simulink model "ME425QuadcoptorMotionControlV4"  (R2024b)
settings: Solver=VariableStepAuto  StartTime=0.0  StopTime=simTime  FixedStep=1e-9  RelTol=1e-2
values from neighbouring files (symbols this model uses):
  D_phi = 0.95    [ME425HW3QuadcoptorMotionControl.m]
  D_psi = 0.95    [ME425HW3QuadcoptorMotionControl.m]
  D_theta = 0.95    [ME425HW3QuadcoptorMotionControl.m]
  D_z = 2    [ME425HW3QuadcoptorMotionControl.m]
  g = 9.81    [ME425HW3QuadcoptorMotionControl.m]
  I_phi = 0.1    [ME425HW3QuadcoptorMotionControl.m]
  I_psi = 0.05    [ME425HW3QuadcoptorMotionControl.m]
  I_theta = 0.1    [ME425HW3QuadcoptorMotionControl.m]
  I_z = 0.1    [ME425HW3QuadcoptorMotionControl.m]
  initialAngles = [0 0 0]    [ME425HW3QuadcoptorMotionControl.m]
  Ix = 0.02    [ME425HW3QuadcoptorMotionControl.m]
  Iy = 0.02    [ME425HW3QuadcoptorMotionControl.m]
  Iz = 0.04    [ME425HW3QuadcoptorMotionControl.m]
  m = 1    [ME425HW3QuadcoptorMotionControl.m]
  P_phi = 0.5    [ME425HW3QuadcoptorMotionControl.m]
  P_psi = 0.5    [ME425HW3QuadcoptorMotionControl.m]
  P_theta = 0.5    [ME425HW3QuadcoptorMotionControl.m]
  P_z = 0.75    [ME425HW3QuadcoptorMotionControl.m]
  zDesired = 2    [ME425HW3QuadcoptorMotionControl.m]
libraries: slpidlib x4
settings Model: Creator=Arda Gencer  LastModifiedBy=Arda Gencer

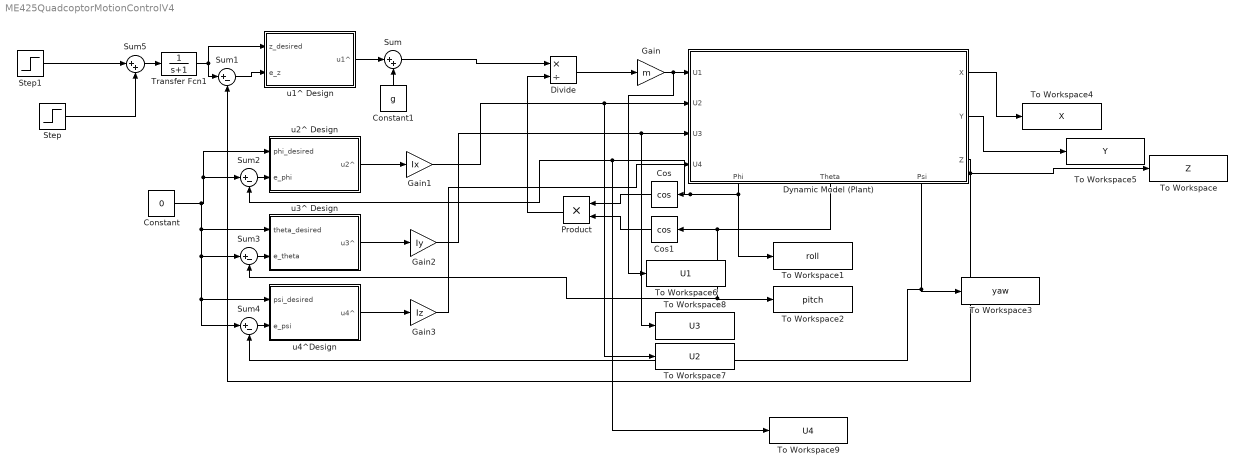
== system ME425QuadcoptorMotionControlV4 ==
  Constant : Constant  Value=0
  Constant1 : Constant  Value=g
  Cos : Trigonometry  Operator=cos
  Cos1 : Trigonometry  Operator=cos
  Divide : Product  Inputs=*/
  Dynamic Model (Plant) : Subsystem
      settings: PortSchema="{\"entries\":[{\"content\":{\"sides\":[{\"content\":{\"connectorIds\":[\"In1\",\"In2\",\"In3\",\"In4\"]},\"type\":\"ConnectorPlacement.EquallySpacedRectSide\",\"uuid\":\"08b1677c-733e-4bff-a275-c4be774b24b5\"},{\"content\":{\"connectorIds\":[\"Out1\",\"Out2\",\"Out3\"],\"side\":\"RIGHT\"},\"type\":\"ConnectorPlacement.EquallySpacedRectSide\",\"uuid\":\"655169e1-9348-4dc0-9050-0d096e576661\"},{\"content\":{\"side\":\"TOP\"},\"type\":\"ConnectorPlacement.EquallySpacedRectSide\",\"uuid\":\"6c01dbd3-88d9-43d1-9966-b2f3dc36f972\"},{\"content\":{\"connectorIds\":[\"Out4\",\"Out5\",\"Out6\"],\"side\":\"BOTTOM\"},\"type\":\"ConnectorPlacement.EquallySpacedRectSide\",\"uuid\":\"d00d5ad9-d72f-434d-885b-77b5f35ca427\"}]},\"type\":\"ConnectorPlacement.EquallySpacedConnector\",\"uuid\":\"87e83324-135b-4426-b2c1-a0cfdb552e41\"}],\"packageUris\":[\"http://schema.mathworks.com/mf0/Connector/R2020b\"],\"version\":\"1.0\"}"
  Gain : Gain  Gain=m
  Gain1 : Gain  Gain=Ix
  Gain2 : Gain  Gain=Iy
  Gain3 : Gain  Gain=Iz
  Product : Product
  Step : Step  Time=0  After=zDesired  SampleTime=0
  Step1 : Step  Time=30  After=-zDesired  SampleTime=0
  Sum : Sum  Inputs=|++
  Sum{1..4} (4 alike) : Sum  Inputs=|+-
  Sum5 : Sum  Inputs=|++
  To Workspace : ToWorkspace  VariableName=Z  SampleTime=-1
  To Workspace1 : ToWorkspace  VariableName=roll  SampleTime=-1
  To Workspace2 : ToWorkspace  VariableName=pitch  SampleTime=-1
  To Workspace3 : ToWorkspace  VariableName=yaw  SampleTime=-1
  To Workspace4 : ToWorkspace  VariableName=X  SampleTime=-1
  To Workspace5 : ToWorkspace  VariableName=Y  SampleTime=-1
  To Workspace6 : ToWorkspace  VariableName=U1  SampleTime=-1
  To Workspace7 : ToWorkspace  VariableName=U2  SampleTime=-1
  To Workspace8 : ToWorkspace  VariableName=U3  SampleTime=-1
  To Workspace9 : ToWorkspace  VariableName=U4  SampleTime=-1
  Transfer Fcn1 : TransferFcn  Denominator=[1 1]
  u1^ Design : Subsystem
  u2^ Design : Subsystem
  u3^ Design : Subsystem
  u4^Design : Subsystem
  wires:
  Dynamic Model (Plant)/3(Z) -> Sum1/2, To Workspace/1
  Dynamic Model (Plant)/4(Phi) -> To Workspace1/1, To Workspace9/1, Sum2/2, Cos/1
  Dynamic Model (Plant)/5(Theta) -> Sum3/2, To Workspace2/1, Cos1/1
  Dynamic Model (Plant)/6(Psi) -> Sum4/2, To Workspace3/1
  Transfer Fcn1/1 -> u1^ Design/1(z_desired), Sum1/1
  Constant1/1 -> Sum/2
  Gain/1 -> To Workspace6/1, Dynamic Model (Plant)/1(U1)
  Divide/1 -> Gain/1
  Product/1 -> Divide/2
  Sum/1 -> Divide/1
  Cos/1 -> Product/1
  Cos1/1 -> Product/2
  u1^ Design/1(u1^) -> Sum/1
  Sum1/1 -> u1^ Design/2(e_z)
  Constant/1 -> Sum4/1, u4^Design/1(psi_desired), Sum3/1, u3^ Design/1(theta_desired), Sum2/1, u2^ Design/1(phi_desired)
  Sum4/1 -> u4^Design/2(e_psi)
  Sum3/1 -> u3^ Design/2(e_theta)
  Sum2/1 -> u2^ Design/2(e_phi)
  u2^ Design/1(u2^) -> Gain1/1
  u4^Design/1(u4^) -> Gain3/1
  u3^ Design/1(u3^) -> Gain2/1
  Gain1/1 -> To Workspace7/1, Dynamic Model (Plant)/2(U2)
  Gain2/1 -> Dynamic Model (Plant)/3(U3), To Workspace8/1
  Gain3/1 -> Dynamic Model (Plant)/4(U4)
  Step1/1 -> Sum5/1
  Step/1 -> Sum5/2
  Dynamic Model (Plant)/1(X) -> To Workspace4/1
  Dynamic Model (Plant)/2(Y) -> To Workspace5/1
  Sum5/1 -> Transfer Fcn1/1

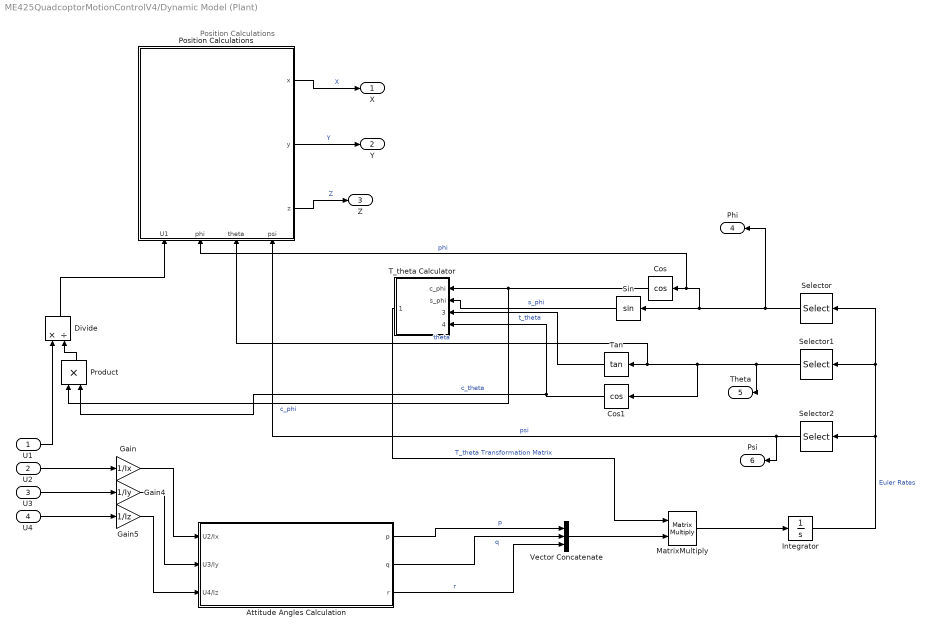
== system ME425QuadcoptorMotionControlV4/Dynamic Model (Plant) ==
  note: Position Calculations
  U1 : Inport
  U2 : Inport  Port=2
  U3 : Inport  Port=3
  U4 : Inport  Port=4
  Attitude Angles Calculation : Subsystem
  Cos : Trigonometry  Operator=cos
  Cos1 : Trigonometry  Operator=cos
  Divide : Product  Inputs=*/
  Gain : Gain  Gain=1/Ix
  Gain4 : Gain  Gain=1/Iy
  Gain5 : Gain  Gain=1/Iz
  Integrator : Integrator  InitialCondition=initialAngles
  MatrixMultiply : Product  Multiplication=Matrix(*)
  Position Calculations : Subsystem
      settings: PortSchema="{\"entries\":[{\"content\":{\"sides\":[{\"content\":{\"connectorIds\":[\"In1\",\"In2\",\"In3\",\"In4\"]},\"type\":\"ConnectorPlacement.EquallySpacedRectSide\",\"uuid\":\"bd898587-7085-4c8a-abc4-67bd8d59ea08\"},{\"content\":{\"side\":\"RIGHT\"},\"type\":\"ConnectorPlacement.EquallySpacedRectSide\",\"uuid\":\"f25e6be6-ac4f-428e-a4d0-66b7114170c6\"},{\"content\":{\"side\":\"TOP\"},\"type\":\"ConnectorPlacement.EquallySpacedRectSide\",\"uuid\":\"1b5079d3-453d-4b69-91fa-2e9092c60c78\"},{\"content\":{\"connectorIds\":[\"Out1\",\"Out2\",\"Out3\"],\"side\":\"BOTTOM\"},\"type\":\"ConnectorPlacement.EquallySpacedRectSide\",\"uuid\":\"956a8f80-6aeb-4d85-a1cd-c5deb734e20d\"}]},\"type\":\"ConnectorPlacement.EquallySpacedConnector\",\"uuid\":\"f46b91c2-157f-4b6c-9de1-eab5cbe73704\"}],\"packageUris\":[\"http://schema.mathworks.com/mf0/Connector/R2020b\"],\"version\":\"1.0\"}"
  Product : Product
  Selector : Selector  InputPortWidth=3  IndexOptions=Index vector (dialog)  Indices=[1]  OutputSizes=1
  Selector1 : Selector  InputPortWidth=3  IndexOptions=Index vector (dialog)  Indices=2  OutputSizes=1
  Selector2 : Selector  InputPortWidth=3  IndexOptions=Index vector (dialog)  Indices=3  OutputSizes=1
  Sin : Trigonometry
  T_theta Calculator : Subsystem
  Tan : Trigonometry  Operator=tan
  Vector Concatenate : Concatenate  NumInputs=3
  X : Outport
  Y : Outport  Port=2
  Z : Outport  Port=3
  Phi : Outport  Port=4
  Theta : Outport  Port=5
  Psi : Outport  Port=6
  wires:
  Vector Concatenate/1 -> MatrixMultiply/2
  Selector1/1 -> Theta/1, Position Calculations/3(theta), Tan/1, Cos1/1  "theta"
  Attitude Angles Calculation/2(q) -> Vector Concatenate/2  "q"
  U4/1 -> Gain5/1
  Cos/1 -> Product/1, T_theta Calculator/1(c_phi)  "c_phi"
  Selector/1 -> Phi/1, Position Calculations/2(phi), Cos/1, Sin/1  "phi"
  Gain/1 -> Attitude Angles Calculation/1(U2/Ix)
  Gain5/1 -> Attitude Angles Calculation/3(U4/Iz)
  Attitude Angles Calculation/3(r) -> Vector Concatenate/3  "r"
  Tan/1 -> T_theta Calculator/3(t_theta)  "t_theta"
  Sin/1 -> T_theta Calculator/2(s_phi)  "s_phi"
  Cos1/1 -> Product/2, T_theta Calculator/4(c_theta)  "c_theta"
  MatrixMultiply/1 -> Integrator/1
  T_theta Calculator/1(T_theta) -> MatrixMultiply/1  "T_theta Transformation Matrix"
  U2/1 -> Gain/1
  U3/1 -> Gain4/1
  Selector2/1 -> Psi/1, Position Calculations/4(psi)  "psi"
  Attitude Angles Calculation/1(p) -> Vector Concatenate/1  "p"
  Position Calculations/1(z) -> Z/1  "Z"
  Gain4/1 -> Attitude Angles Calculation/2(U3/Iy)
  Position Calculations/3(x) -> X/1  "X"
  Position Calculations/2(y) -> Y/1  "Y"
  U1/1 -> Divide/1
  Divide/1 -> Position Calculations/1(U1)
  Product/1 -> Divide/2
  Integrator/1 -> Selector/1, Selector1/1, Selector2/1  "Euler Rates"

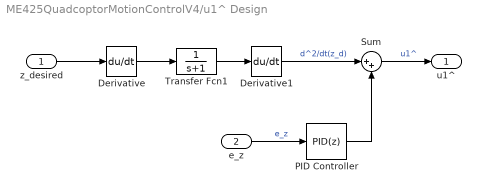
== system ME425QuadcoptorMotionControlV4/u1^ Design ==
  z_desired : Inport
  e_z : Inport  Port=2
  Derivative : Derivative
  Derivative1 : Derivative
  PID Controller : slpidlib/PID Controller  Controller=PID  Form=Parallel  TimeDomain=Discrete-time  UseExternalTs=off  SampleTime=0.001  IntegratorMethod=Forward Euler  FilterMethod=Forward Euler  ControllerParametersSource=internal  P=P_z  I=I_z  UseKiTs=off  D=D_z  UseExternalDerivativeSource=off  N=100  UseFilter=on  TunerSelectOption=Transfer Function Based (PID Tuner App)  InitialConditionSource=internal  InitialConditionForIntegrator=0  InitialConditionForFilter=0  DifferentiatorICPrevScaledInput=0  ExternalReset=none  TrackingMode=off  Kt=1  LimitOutput=off  SatLimitsSource=internal  UpperSaturationLimit=inf  LowerSaturationLimit=-inf  LinearizeAsGain=on  AntiWindupMode=none  Kb=1  LimitIntegrator=off  UpperIntegratorSaturationLimit=inf  LowerIntegratorSaturationLimit=-inf  POutMin=[]  POutMax=[]  IOutMin=[]  IOutMax=[]  DOutMin=[]  DOutMax=[]  NOutMin=[]  NOutMax=[]  SumOutMin=[]  SumOutMax=[]  SaturationOutMin=[]  SaturationOutMax=[]  PParamMin=[]  PParamMax=[]  IParamMin=[]  IParamMax=[]  DParamMin=[]  DParamMax=[]  NParamMin=[]  NParamMax=[]  KbParamMin=[]  KbParamMax=[]  KtParamMin=[]  KtParamMax=[]  KbOutMin=[]  KbOutMax=[]  KtOutMin=[]  KtOutMax=[]  IntegratorOutMin=[]  IntegratorOutMax=[]  FilterOutMin=[]  FilterOutMax=[]  SumI1OutMin=[]  SumI1OutMax=[]  SumI2OutMin=[]  SumI2OutMax=[]  SumI3OutMin=[]  SumI3OutMax=[]  SumI4OutMin=[]  SumI4OutMax=[]  SumDOutMin=[]  SumDOutMax=[]  DifferentiatorOutMin=[]  DifferentiatorOutMax=[]  FilterDiffOutCoefMin=[]  FilterDiffOutCoefMax=[]  ReciprocalOutMin=[]  ReciprocalOutMax=[]  SumDenOutMin=[]  SumDenOutMax=[]  SumNumOutMin=[]  SumNumOutMax=[]  DivideOutMin=[]  DivideOutMax=[]  UdiffTsProdOutMin=[]  UdiffTsProdOutMax=[]  NTsProdOutMin=[]  NTsProdOutMax=[]  UintegralTsProdOutMin=[]  UintegralTsProdOutMax=[]  UngainTsProdOutMin=[]  UngainTsProdOutMax=[]  ClampingZeroOutDataTypeStr=Inherit: Inherit via back propagation  ClampingZeroOutMin=[]  ClampingZeroOutMax=[]  FilterDenConstantOutDataTypeStr=Inherit: Inherit via back propagation  FilterDenConstantOutMin=[]  FilterDenConstantOutMax=[]  PCopyOutDataTypeStr=Inherit: Inherit via back propagation  PCopyOutMin=[]  PCopyOutMax=[]  NCopyOutDataTypeStr=Inherit: Inherit via back propagation  NCopyOutMin=[]  NCopyOutMax=[]  IntegratorContinuousStateAttributes=''  IntegratorStateMustResolveToSignalObject=off  IntegratorRTWStateStorageClass=Auto  FilterContinuousStateAttributes=''  FilterStateMustResolveToSignalObject=off  FilterRTWStateStorageClass=Auto  ParallelPVariant=InternalParameters  IdealPVariant=Disabled  IVariant=InternalParameters  DVariant=InternalParameters  IntegratorVariant=Discrete  SatVariant=Disabled  AWVariant=Passthrough  PCopyVariant=Disabled  TRVariant=Disabled  FdbkBlocksVariant=Forward  IdealPFdbkVariant=Disabled  SatFdbkVariant=Disabled  DerivativeFilterVariant=ForwardEulerFilter  NVariant=InternalParameters  NCopyVariant=Disabled  FilterICVariant=InternalICsFilter  IntegratorICVariant=InternalICs  ExternalResetVariant=Disabled  TRSumVariant=Passthrough  SumFdbkVariant=Disabled  SumVariant=Sum_PID  TsampFilterVariant=InternalTs  TsampNgainVariant=Passthrough  TsampIntegralVariant=Disabled_SignalSpec  ExternalSaturationOutDataTypeStr=Inherit: Same as second input  DerivativeSourceVariant=ErrorSignal  PreIntVariant=InternalPreInt
  Sum : Sum  Inputs=|++
  Transfer Fcn1 : TransferFcn  Denominator=[1 1]
  u1^ : Outport
  wires:
  z_desired/1 -> Derivative/1
  Derivative1/1 -> Sum/1  "d^2/dt(z_d)"
  Derivative/1 -> Transfer Fcn1/1
  PID Controller/1 -> Sum/2
  e_z/1 -> PID Controller/1  "e_z"
  Sum/1 -> u1^/1  "u1^"
  Transfer Fcn1/1 -> Derivative1/1

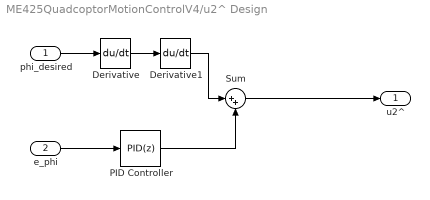
== system ME425QuadcoptorMotionControlV4/u2^ Design ==
  phi_desired : Inport
  e_phi : Inport  Port=2
  Derivative : Derivative
  Derivative1 : Derivative
  PID Controller : slpidlib/PID Controller  Controller=PID  Form=Parallel  TimeDomain=Discrete-time  UseExternalTs=off  SampleTime=0.001  IntegratorMethod=Forward Euler  FilterMethod=Forward Euler  ControllerParametersSource=internal  P=P_phi  I=I_phi  UseKiTs=off  D=D_phi  UseExternalDerivativeSource=off  N=100  UseFilter=on  TunerSelectOption=Transfer Function Based (PID Tuner App)  InitialConditionSource=internal  InitialConditionForIntegrator=0  InitialConditionForFilter=0  DifferentiatorICPrevScaledInput=0  ExternalReset=none  TrackingMode=off  Kt=1  LimitOutput=off  SatLimitsSource=internal  UpperSaturationLimit=inf  LowerSaturationLimit=-inf  LinearizeAsGain=on  AntiWindupMode=none  Kb=1  LimitIntegrator=off  UpperIntegratorSaturationLimit=inf  LowerIntegratorSaturationLimit=-inf  POutMin=[]  POutMax=[]  IOutMin=[]  IOutMax=[]  DOutMin=[]  DOutMax=[]  NOutMin=[]  NOutMax=[]  SumOutMin=[]  SumOutMax=[]  SaturationOutMin=[]  SaturationOutMax=[]  PParamMin=[]  PParamMax=[]  IParamMin=[]  IParamMax=[]  DParamMin=[]  DParamMax=[]  NParamMin=[]  NParamMax=[]  KbParamMin=[]  KbParamMax=[]  KtParamMin=[]  KtParamMax=[]  KbOutMin=[]  KbOutMax=[]  KtOutMin=[]  KtOutMax=[]  IntegratorOutMin=[]  IntegratorOutMax=[]  FilterOutMin=[]  FilterOutMax=[]  SumI1OutMin=[]  SumI1OutMax=[]  SumI2OutMin=[]  SumI2OutMax=[]  SumI3OutMin=[]  SumI3OutMax=[]  SumI4OutMin=[]  SumI4OutMax=[]  SumDOutMin=[]  SumDOutMax=[]  DifferentiatorOutMin=[]  DifferentiatorOutMax=[]  FilterDiffOutCoefMin=[]  FilterDiffOutCoefMax=[]  ReciprocalOutMin=[]  ReciprocalOutMax=[]  SumDenOutMin=[]  SumDenOutMax=[]  SumNumOutMin=[]  SumNumOutMax=[]  DivideOutMin=[]  DivideOutMax=[]  UdiffTsProdOutMin=[]  UdiffTsProdOutMax=[]  NTsProdOutMin=[]  NTsProdOutMax=[]  UintegralTsProdOutMin=[]  UintegralTsProdOutMax=[]  UngainTsProdOutMin=[]  UngainTsProdOutMax=[]  ClampingZeroOutDataTypeStr=Inherit: Inherit via back propagation  ClampingZeroOutMin=[]  ClampingZeroOutMax=[]  FilterDenConstantOutDataTypeStr=Inherit: Inherit via back propagation  FilterDenConstantOutMin=[]  FilterDenConstantOutMax=[]  PCopyOutDataTypeStr=Inherit: Inherit via back propagation  PCopyOutMin=[]  PCopyOutMax=[]  NCopyOutDataTypeStr=Inherit: Inherit via back propagation  NCopyOutMin=[]  NCopyOutMax=[]  IntegratorContinuousStateAttributes=''  IntegratorStateMustResolveToSignalObject=off  IntegratorRTWStateStorageClass=Auto  FilterContinuousStateAttributes=''  FilterStateMustResolveToSignalObject=off  FilterRTWStateStorageClass=Auto  ParallelPVariant=InternalParameters  IdealPVariant=Disabled  IVariant=InternalParameters  DVariant=InternalParameters  IntegratorVariant=Discrete  SatVariant=Disabled  AWVariant=Passthrough  PCopyVariant=Disabled  TRVariant=Disabled  FdbkBlocksVariant=Forward  IdealPFdbkVariant=Disabled  SatFdbkVariant=Disabled  DerivativeFilterVariant=ForwardEulerFilter  NVariant=InternalParameters  NCopyVariant=Disabled  FilterICVariant=InternalICsFilter  IntegratorICVariant=InternalICs  ExternalResetVariant=Disabled  TRSumVariant=Passthrough  SumFdbkVariant=Disabled  SumVariant=Sum_PID  TsampFilterVariant=InternalTs  TsampNgainVariant=Passthrough  TsampIntegralVariant=Disabled_SignalSpec  ExternalSaturationOutDataTypeStr=Inherit: Same as second input  DerivativeSourceVariant=ErrorSignal  PreIntVariant=InternalPreInt
  Sum : Sum  Inputs=|++
  u2^ : Outport
  wires:
  phi_desired/1 -> Derivative/1
  Derivative/1 -> Derivative1/1
  e_phi/1 -> PID Controller/1
  Derivative1/1 -> Sum/1
  PID Controller/1 -> Sum/2
  Sum/1 -> u2^/1

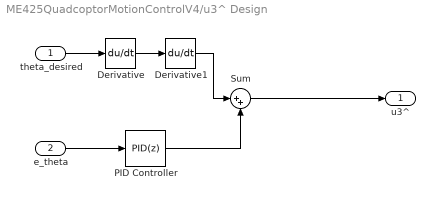
== system ME425QuadcoptorMotionControlV4/u3^ Design ==
  theta_desired : Inport
  e_theta : Inport  Port=2
  Derivative : Derivative
  Derivative1 : Derivative
  PID Controller : slpidlib/PID Controller  Controller=PID  Form=Parallel  TimeDomain=Discrete-time  UseExternalTs=off  SampleTime=0.001  IntegratorMethod=Forward Euler  FilterMethod=Forward Euler  ControllerParametersSource=internal  P=P_theta  I=I_theta  UseKiTs=off  D=D_theta  UseExternalDerivativeSource=off  N=100  UseFilter=on  TunerSelectOption=Transfer Function Based (PID Tuner App)  InitialConditionSource=internal  InitialConditionForIntegrator=0  InitialConditionForFilter=0  DifferentiatorICPrevScaledInput=0  ExternalReset=none  TrackingMode=off  Kt=1  LimitOutput=off  SatLimitsSource=internal  UpperSaturationLimit=inf  LowerSaturationLimit=-inf  LinearizeAsGain=on  AntiWindupMode=none  Kb=1  LimitIntegrator=off  UpperIntegratorSaturationLimit=inf  LowerIntegratorSaturationLimit=-inf  POutMin=[]  POutMax=[]  IOutMin=[]  IOutMax=[]  DOutMin=[]  DOutMax=[]  NOutMin=[]  NOutMax=[]  SumOutMin=[]  SumOutMax=[]  SaturationOutMin=[]  SaturationOutMax=[]  PParamMin=[]  PParamMax=[]  IParamMin=[]  IParamMax=[]  DParamMin=[]  DParamMax=[]  NParamMin=[]  NParamMax=[]  KbParamMin=[]  KbParamMax=[]  KtParamMin=[]  KtParamMax=[]  KbOutMin=[]  KbOutMax=[]  KtOutMin=[]  KtOutMax=[]  IntegratorOutMin=[]  IntegratorOutMax=[]  FilterOutMin=[]  FilterOutMax=[]  SumI1OutMin=[]  SumI1OutMax=[]  SumI2OutMin=[]  SumI2OutMax=[]  SumI3OutMin=[]  SumI3OutMax=[]  SumI4OutMin=[]  SumI4OutMax=[]  SumDOutMin=[]  SumDOutMax=[]  DifferentiatorOutMin=[]  DifferentiatorOutMax=[]  FilterDiffOutCoefMin=[]  FilterDiffOutCoefMax=[]  ReciprocalOutMin=[]  ReciprocalOutMax=[]  SumDenOutMin=[]  SumDenOutMax=[]  SumNumOutMin=[]  SumNumOutMax=[]  DivideOutMin=[]  DivideOutMax=[]  UdiffTsProdOutMin=[]  UdiffTsProdOutMax=[]  NTsProdOutMin=[]  NTsProdOutMax=[]  UintegralTsProdOutMin=[]  UintegralTsProdOutMax=[]  UngainTsProdOutMin=[]  UngainTsProdOutMax=[]  ClampingZeroOutDataTypeStr=Inherit: Inherit via back propagation  ClampingZeroOutMin=[]  ClampingZeroOutMax=[]  FilterDenConstantOutDataTypeStr=Inherit: Inherit via back propagation  FilterDenConstantOutMin=[]  FilterDenConstantOutMax=[]  PCopyOutDataTypeStr=Inherit: Inherit via back propagation  PCopyOutMin=[]  PCopyOutMax=[]  NCopyOutDataTypeStr=Inherit: Inherit via back propagation  NCopyOutMin=[]  NCopyOutMax=[]  IntegratorContinuousStateAttributes=''  IntegratorStateMustResolveToSignalObject=off  IntegratorRTWStateStorageClass=Auto  FilterContinuousStateAttributes=''  FilterStateMustResolveToSignalObject=off  FilterRTWStateStorageClass=Auto  ParallelPVariant=InternalParameters  IdealPVariant=Disabled  IVariant=InternalParameters  DVariant=InternalParameters  IntegratorVariant=Discrete  SatVariant=Disabled  AWVariant=Passthrough  PCopyVariant=Disabled  TRVariant=Disabled  FdbkBlocksVariant=Forward  IdealPFdbkVariant=Disabled  SatFdbkVariant=Disabled  DerivativeFilterVariant=ForwardEulerFilter  NVariant=InternalParameters  NCopyVariant=Disabled  FilterICVariant=InternalICsFilter  IntegratorICVariant=InternalICs  ExternalResetVariant=Disabled  TRSumVariant=Passthrough  SumFdbkVariant=Disabled  SumVariant=Sum_PID  TsampFilterVariant=InternalTs  TsampNgainVariant=Passthrough  TsampIntegralVariant=Disabled_SignalSpec  ExternalSaturationOutDataTypeStr=Inherit: Same as second input  DerivativeSourceVariant=ErrorSignal  PreIntVariant=InternalPreInt
  Sum : Sum  Inputs=|++
  u3^ : Outport
  wires:
  theta_desired/1 -> Derivative/1
  Derivative/1 -> Derivative1/1
  e_theta/1 -> PID Controller/1
  Derivative1/1 -> Sum/1
  PID Controller/1 -> Sum/2
  Sum/1 -> u3^/1

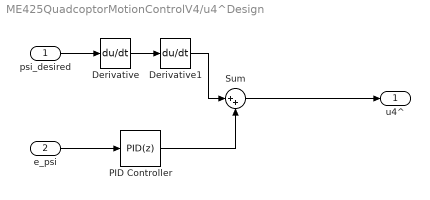
== system ME425QuadcoptorMotionControlV4/u4^Design ==
  psi_desired : Inport
  e_psi : Inport  Port=2
  Derivative : Derivative
  Derivative1 : Derivative
  PID Controller : slpidlib/PID Controller  Controller=PID  Form=Parallel  TimeDomain=Discrete-time  UseExternalTs=off  SampleTime=0.001  IntegratorMethod=Forward Euler  FilterMethod=Forward Euler  ControllerParametersSource=internal  P=P_psi  I=I_psi  UseKiTs=off  D=D_psi  UseExternalDerivativeSource=off  N=100  UseFilter=on  TunerSelectOption=Transfer Function Based (PID Tuner App)  InitialConditionSource=internal  InitialConditionForIntegrator=0  InitialConditionForFilter=0  DifferentiatorICPrevScaledInput=0  ExternalReset=none  TrackingMode=off  Kt=1  LimitOutput=off  SatLimitsSource=internal  UpperSaturationLimit=inf  LowerSaturationLimit=-inf  LinearizeAsGain=on  AntiWindupMode=none  Kb=1  LimitIntegrator=off  UpperIntegratorSaturationLimit=inf  LowerIntegratorSaturationLimit=-inf  POutMin=[]  POutMax=[]  IOutMin=[]  IOutMax=[]  DOutMin=[]  DOutMax=[]  NOutMin=[]  NOutMax=[]  SumOutMin=[]  SumOutMax=[]  SaturationOutMin=[]  SaturationOutMax=[]  PParamMin=[]  PParamMax=[]  IParamMin=[]  IParamMax=[]  DParamMin=[]  DParamMax=[]  NParamMin=[]  NParamMax=[]  KbParamMin=[]  KbParamMax=[]  KtParamMin=[]  KtParamMax=[]  KbOutMin=[]  KbOutMax=[]  KtOutMin=[]  KtOutMax=[]  IntegratorOutMin=[]  IntegratorOutMax=[]  FilterOutMin=[]  FilterOutMax=[]  SumI1OutMin=[]  SumI1OutMax=[]  SumI2OutMin=[]  SumI2OutMax=[]  SumI3OutMin=[]  SumI3OutMax=[]  SumI4OutMin=[]  SumI4OutMax=[]  SumDOutMin=[]  SumDOutMax=[]  DifferentiatorOutMin=[]  DifferentiatorOutMax=[]  FilterDiffOutCoefMin=[]  FilterDiffOutCoefMax=[]  ReciprocalOutMin=[]  ReciprocalOutMax=[]  SumDenOutMin=[]  SumDenOutMax=[]  SumNumOutMin=[]  SumNumOutMax=[]  DivideOutMin=[]  DivideOutMax=[]  UdiffTsProdOutMin=[]  UdiffTsProdOutMax=[]  NTsProdOutMin=[]  NTsProdOutMax=[]  UintegralTsProdOutMin=[]  UintegralTsProdOutMax=[]  UngainTsProdOutMin=[]  UngainTsProdOutMax=[]  ClampingZeroOutDataTypeStr=Inherit: Inherit via back propagation  ClampingZeroOutMin=[]  ClampingZeroOutMax=[]  FilterDenConstantOutDataTypeStr=Inherit: Inherit via back propagation  FilterDenConstantOutMin=[]  FilterDenConstantOutMax=[]  PCopyOutDataTypeStr=Inherit: Inherit via back propagation  PCopyOutMin=[]  PCopyOutMax=[]  NCopyOutDataTypeStr=Inherit: Inherit via back propagation  NCopyOutMin=[]  NCopyOutMax=[]  IntegratorContinuousStateAttributes=''  IntegratorStateMustResolveToSignalObject=off  IntegratorRTWStateStorageClass=Auto  FilterContinuousStateAttributes=''  FilterStateMustResolveToSignalObject=off  FilterRTWStateStorageClass=Auto  ParallelPVariant=InternalParameters  IdealPVariant=Disabled  IVariant=InternalParameters  DVariant=InternalParameters  IntegratorVariant=Discrete  SatVariant=Disabled  AWVariant=Passthrough  PCopyVariant=Disabled  TRVariant=Disabled  FdbkBlocksVariant=Forward  IdealPFdbkVariant=Disabled  SatFdbkVariant=Disabled  DerivativeFilterVariant=ForwardEulerFilter  NVariant=InternalParameters  NCopyVariant=Disabled  FilterICVariant=InternalICsFilter  IntegratorICVariant=InternalICs  ExternalResetVariant=Disabled  TRSumVariant=Passthrough  SumFdbkVariant=Disabled  SumVariant=Sum_PID  TsampFilterVariant=InternalTs  TsampNgainVariant=Passthrough  TsampIntegralVariant=Disabled_SignalSpec  ExternalSaturationOutDataTypeStr=Inherit: Same as second input  DerivativeSourceVariant=ErrorSignal  PreIntVariant=InternalPreInt
  Sum : Sum  Inputs=|++
  u4^ : Outport
  wires:
  psi_desired/1 -> Derivative/1
  Derivative/1 -> Derivative1/1
  e_psi/1 -> PID Controller/1
  Derivative1/1 -> Sum/1
  PID Controller/1 -> Sum/2
  Sum/1 -> u4^/1

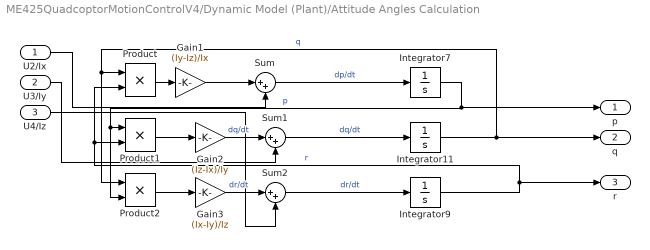
== system ME425QuadcoptorMotionControlV4/Dynamic Model (Plant)/Attitude Angles Calculation ==
  U2/Ix : Inport
  U3/Iy : Inport  Port=2
  U4/Iz : Inport  Port=3
  Gain1 : Gain  Gain=(Iy-Iz)/Ix
  Gain2 : Gain  Gain=(Iz-Ix)/Iy
  Gain3 : Gain  Gain=(Ix-Iy)/Iz
  Integrator11 : Integrator
  Integrator7 : Integrator
  Integrator9 : Integrator
  Product : Product
  Product1 : Product
  Product2 : Product
  Sum : Sum  Inputs=|++
  Sum1 : Sum  Inputs=|++
  Sum2 : Sum  Inputs=|++
  p : Outport
  q : Outport  Port=2
  r : Outport  Port=3
  wires:
  Integrator11/1 -> q/1, Product2/1, Product/1  "q"
  Integrator7/1 -> Product2/2, Product1/1, p/1  "p"
  Gain1/1 -> Sum/1
  Integrator9/1 -> Product1/2, Product/2, r/1  "r"
  Product2/1 -> Gain3/1
  Sum/1 -> Integrator7/1  "dp/dt"
  Product1/1 -> Gain2/1
  Gain2/1 -> Sum1/1  "dq/dt"
  Gain3/1 -> Sum2/1  "dr/dt"
  Sum1/1 -> Integrator11/1  "dq/dt"
  Sum2/1 -> Integrator9/1  "dr/dt"
  U3/Iy/1 -> Sum1/2
  Product/1 -> Gain1/1
  U2/Ix/1 -> Sum/2
  U4/Iz/1 -> Sum2/2

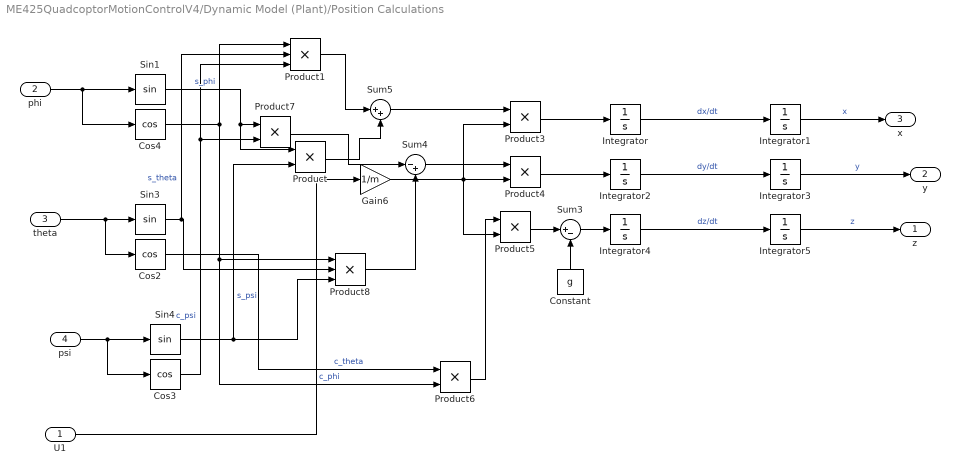
== system ME425QuadcoptorMotionControlV4/Dynamic Model (Plant)/Position Calculations ==
  U1 : Inport
  phi : Inport  Port=2
  theta : Inport  Port=3
  psi : Inport  Port=4
  Constant : Constant  Value=g
  Cos2 : Trigonometry  Operator=cos
  Cos3 : Trigonometry  Operator=cos
  Cos4 : Trigonometry  Operator=cos
  Gain6 : Gain  Gain=1/m
  Integrator{,1..5} (6 alike) : Integrator
  Product{,3..7} (6 alike) : Product
  Product1 : Product  Inputs=3
  Product8 : Product  Inputs=3
  Sin1 : Trigonometry
  Sin3 : Trigonometry
  Sin4 : Trigonometry
  Sum3 : Sum  Inputs=|+-
  Sum4 : Sum  Inputs=|-+
  Sum5 : Sum  Inputs=|++
  z : Outport
  y : Outport  Port=2
  x : Outport  Port=3
  wires:
  Integrator4/1 -> Integrator5/1  "dz/dt"
  Sin3/1 -> Product1/2, Product8/2  "s_theta"
  psi/1 -> Cos3/1, Sin4/1
  U1/1 -> Gain6/1
  Sum4/1 -> Product4/1
  Integrator2/1 -> Integrator3/1  "dy/dt"
  Cos4/1 -> Product8/1, Product6/2, Product1/1  "c_phi"
  Integrator1/1 -> x/1  "x"
  theta/1 -> Cos2/1, Sin3/1
  Gain6/1 -> Product3/2, Product5/2, Product4/2
  Sum3/1 -> Integrator4/1
  Sin4/1 -> Product/2, Product8/3  "s_psi"
  Product1/1 -> Sum5/1
  Integrator/1 -> Integrator1/1  "dx/dt"
  Sum5/1 -> Product3/1
  Cos3/1 -> Product1/3, Product7/2  "c_psi"
  Product3/1 -> Integrator/1
  Product4/1 -> Integrator2/1
  Cos2/1 -> Product6/1  "c_theta"
  phi/1 -> Cos4/1, Sin1/1
  Product7/1 -> Sum4/1
  Product6/1 -> Product5/1
  Product/1 -> Sum5/2
  Constant/1 -> Sum3/2
  Product5/1 -> Sum3/1
  Sin1/1 -> Product/1, Product7/1  "s_phi"
  Product8/1 -> Sum4/2
  Integrator3/1 -> y/1  "y"
  Integrator5/1 -> z/1  "z"

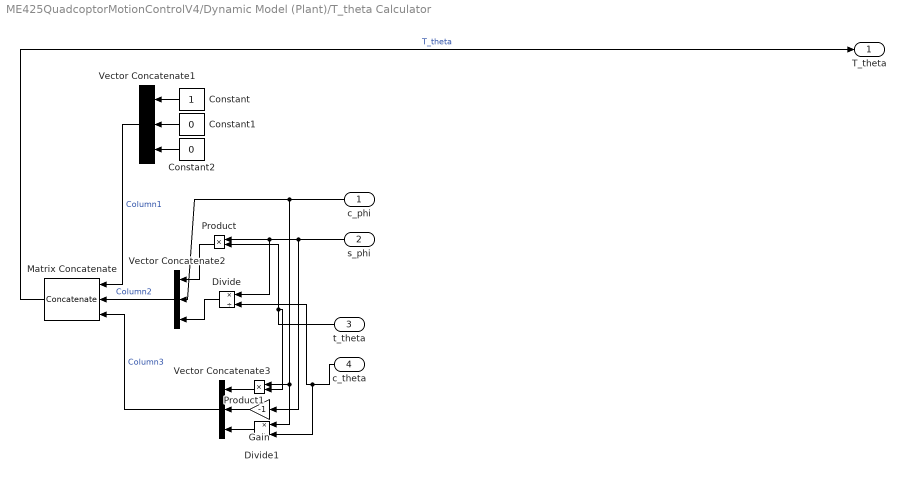
== system ME425QuadcoptorMotionControlV4/Dynamic Model (Plant)/T_theta Calculator ==
  c_phi : Inport
  s_phi : Inport  Port=2
  t_theta : Inport  Port=3
  c_theta : Inport  Port=4
  Constant : Constant
  Constant1 : Constant  Value=0
  Constant2 : Constant  Value=0
  Divide : Product  Inputs=*/
  Divide1 : Product  Inputs=*/
  Gain : Gain  Gain=-1
  Matrix Concatenate : Concatenate  NumInputs=3  Mode=Multidimensional array  ConcatenateDimension=2
  Product : Product
  Product1 : Product
  Vector Concatenate1 : Concatenate  NumInputs=3
  Vector Concatenate2 : Concatenate  NumInputs=3
  Vector Concatenate3 : Concatenate  NumInputs=3
  T_theta : Outport
  wires:
  c_theta/1 -> Divide/2, Divide1/2
  c_phi/1 -> Vector Concatenate2/2, Divide1/1, Product1/1
  Constant/1 -> Vector Concatenate1/1
  Vector Concatenate2/1 -> Matrix Concatenate/2  "Column2"
  Product/1 -> Vector Concatenate2/1
  s_phi/1 -> Product/1, Divide/1, Gain/1
  Product1/1 -> Vector Concatenate3/1
  Vector Concatenate3/1 -> Matrix Concatenate/3  "Column3"
  Matrix Concatenate/1 -> T_theta/1  "T_theta"
  Constant2/1 -> Vector Concatenate1/3
  Constant1/1 -> Vector Concatenate1/2
  Vector Concatenate1/1 -> Matrix Concatenate/1  "Column1"
  t_theta/1 -> Product1/2, Product/2
  Gain/1 -> Vector Concatenate3/2
  Divide1/1 -> Vector Concatenate3/3
  Divide/1 -> Vector Concatenate2/3
